simulink model "rlc_diode_sps_sl"  (R2014a)
settings: Solver=ode23tb  StartTime=0.0  StopTime=1  MaxStep=0.1  RelTol=1e-4
PreLoadFcn:
  | Vs = 30;
  | L = 1e-3;
  | C = 1e-3;
  | R = 1;
  | sys=power_analyze('rlc_diode_sps','structure');
libraries: powerlib x9
settings Model: Creator=gdudgeon  LastModifiedBy=cosorio
settings DataIOCC: SignalLoggingSaveFormat=ModelDataLogs  SaveTime=off
settings OptimizationCC: ExpressionDepthLimit=2147483647
settings DebuggingCC: UnderspecifiedInitializationDetection=Classic  FcnCallInpInsideContextMsg=UseLocalSettings  StateNameClashWarn=warning
settings GRTTargetCC: CombineOutputUpdateFcns=off  GRTInterface=on

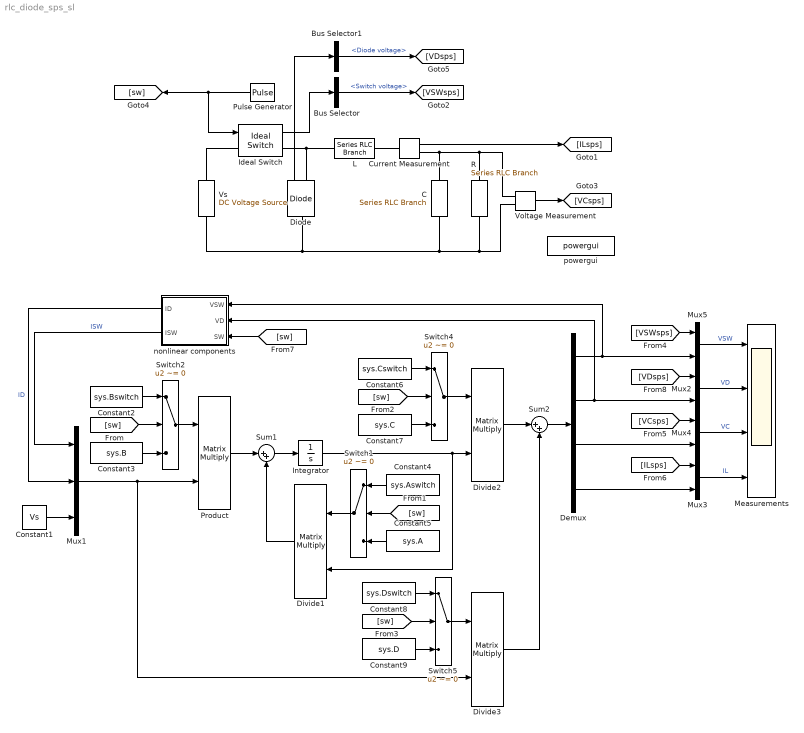
== system rlc_diode_sps_sl ==
  Bus Selector : BusSelector  OutputSignals=Switch voltage
  Bus Selector1 : BusSelector  OutputSignals=Diode voltage
  C : powerlib/Elements/Series RLC Branch  LConnTagsString=__new0  RConnTagsString=__new0  BranchType=C  Resistance=R  Inductance=1e-3  SetiL0=off  InitialCurrent=0  Capacitance=C  Setx0=off  InitialVoltage=0  Measurements=None
  Constant1 : Constant  Value=Vs
  Constant2 : Constant  Value=sys.Bswitch  VectorParams1D=off
  Constant3 : Constant  Value=sys.B  VectorParams1D=off
  Constant4 : Constant  Value=sys.Aswitch
  Constant5 : Constant  Value=sys.A
  Constant6 : Constant  Value=sys.Cswitch
  Constant7 : Constant  Value=sys.C
  Constant8 : Constant  Value=sys.Dswitch
  Constant9 : Constant  Value=sys.D
  Current Measurement : powerlib/Measurements/Current Measurement  PhasorSimulation=off  OutputType=Complex  PSBequivalent=0
  Demux : Demux
  Diode : powerlib/Power Electronics/Diode  Ron=0.001  Lon=0  Vf=0  IC=0  UseSnubber=off  Rs=1e5  Cs=Inf  Measurements=on
  Divide1 : Product  Multiplication=Matrix(*)
  Divide2 : Product  Multiplication=Matrix(*)
  Divide3 : Product  Multiplication=Matrix(*)
  Ideal Switch : powerlib/Power Electronics/Ideal Switch  Ron=0.001  Lon=0  IC=1  Rs=1e5  Cs=inf  Measurements=on
  Integrator : Integrator  InitialCondition=sys.x0
  L : powerlib/Elements/Series RLC Branch  LConnTagsString=__new0  RConnTagsString=__new0  BranchType=L  Resistance=1  Inductance=L  SetiL0=off  InitialCurrent=0  Capacitance=1e-6  Setx0=off  InitialVoltage=0  Measurements=None
  Measurements : Scope  NumInputPorts=4
      settings: YMin=0~-40~0~0  YMax=40~0~20~20
  Mux1 : Mux  Inputs=3
  Mux{2..5} (4 alike) : Mux  Inputs=2
  Product : Product  Multiplication=Matrix(*)  RndMeth=Zero
  Pulse Generator : DiscretePulseGenerator  PulseType=Time based  Period=1e-3  PulseWidth=50
  R : powerlib/Elements/Series RLC Branch  LConnTagsString=__new0  RConnTagsString=__new0  BranchType=R  Resistance=R  Inductance=1e-3  SetiL0=off  InitialCurrent=0  Capacitance=1e-6  Setx0=off  InitialVoltage=0  Measurements=None
  Sum1 : Sum  Inputs=|++
  Sum2 : Sum  Inputs=|++
  Switch{1..2,4..5} (4 alike) : Switch  Criteria=u2 ~= 0  Threshold=0.5
  Voltage Measurement : powerlib/Measurements/Voltage Measurement  PhasorSimulation=off  OutputType=Complex  PSBequivalent=0
  Vs : powerlib/Electrical Sources/DC Voltage Source  Amplitude=Vs  Measurements=None
  nonlinear components : Subsystem
  powergui : powerlib/powergui  SimulationMode=Continuous  SolverType=Tustin  SampleTime=50e-6  frequency=60  SPID=off  DisableSnubberDevices=off  DisableRonSwitches=off  DisableVfSwitches=off  SwTol=0  Interpol=off  DisplayEquations=off  Ts=0  methode=off  frequencyindice=0  Pbase=100e6  ErrMax=1e-4  Iterations=50  UnitsV=kV  UnitsW=MW  FunctionMessages=off  echomessages=off  HookPort=off  EnableUseOfTLC=off  x0status=blocks  RestoreLinks=warning  ResistiveCurrentMeasurement=off  Frange=[0:2:500]  Ylog=off  Xlog=on  ShowGrid=off  save=off  variable=ZData  structure=0  ZoomFFT=on  StartTime=0.0  cycles=1  DisplayStyle=1  fundamental=60  FreqAxis=off  MaxFrequency=1000  frequencyindicesteady=1  RmsSteady=1  display=off
  wires:
  Current Measurement/1 -> [ILsps]
  Voltage Measurement/1 -> [VCsps]
  Pulse Generator/1 -> Ideal Switch/1, [sw]
  Sum2/1 -> Demux/1
  Product/1 -> Sum1/1
  Sum1/1 -> Integrator/1
  Integrator/1 -> Divide2/2, Divide1/2
  [sw] -> Switch1/2
  Constant4/1 -> Switch1/1
  Constant5/1 -> Switch1/3
  [sw] -> Switch4/2
  Constant7/1 -> Switch4/3
  Switch4/1 -> Divide2/1
  Divide2/1 -> Sum2/1
  Divide3/1 -> Sum2/2
  [sw] -> Switch5/2
  Constant8/1 -> Switch5/1
  Constant9/1 -> Switch5/3
  Switch5/1 -> Divide3/1
  nonlinear components/2(ISW) -> Mux1/1  "ISW"
  Constant6/1 -> Switch4/1
  Demux/1 -> Mux5/2, nonlinear components/1(VSW)
  [VSWsps] -> Mux5/1
  [VCsps] -> Mux4/1
  [ILsps] -> Mux3/1
  Mux1/1 -> Product/2, Divide3/2
  Constant3/1 -> Switch2/3
  Switch2/1 -> Product/1
  Constant2/1 -> Switch2/1
  [sw] -> Switch2/2
  Mux5/1 -> Measurements/1  "VSW"
  Divide1/1 -> Sum1/2
  Switch1/1 -> Divide1/1
  Ideal Switch/1 -> Bus Selector/1
  Bus Selector/1 -> [VSWsps]  "<Switch voltage>"
  Constant1/1 -> Mux1/3
  nonlinear components/1(ID) -> Mux1/2  "ID"
  Demux/4 -> Mux3/2
  Demux/3 -> Mux4/2
  Mux3/1 -> Measurements/4  "IL"
  Mux4/1 -> Measurements/3  "VC"
  Mux2/1 -> Measurements/2  "VD"
  [VDsps] -> Mux2/1
  Demux/2 -> nonlinear components/2(VD), Mux2/2
  Diode/1 -> Bus Selector1/1
  Bus Selector1/1 -> [VDsps]  "<Diode voltage>"
  [sw] -> nonlinear components/3(SW)
  connections:
  L/RConn1 -- Current Measurement/LConn1
  Current Measurement/RConn1 -- C/LConn1 -- R/LConn1 -- Voltage Measurement/LConn1
  R/RConn1 -- Voltage Measurement/LConn2 -- C/RConn1 -- Vs/LConn1 -- Diode/LConn1
  Ideal Switch/RConn1 -- L/LConn1 -- Diode/RConn1
  Ideal Switch/LConn1 -- Vs/RConn1

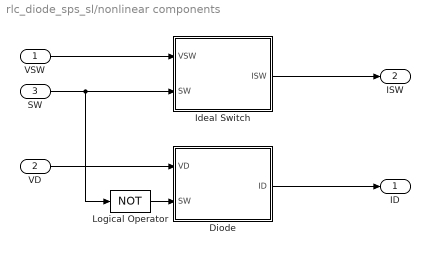
== system rlc_diode_sps_sl/nonlinear components ==
  VSW : Inport
  VD : Inport  Port=2
  SW : Inport  Port=3
  Diode : Subsystem
  Ideal Switch : Subsystem
  Logical Operator : Logic  Operator=NOT  AllPortsSameDT=off  OutDataTypeStr=boolean
  ID : Outport
  ISW : Outport  Port=2
  wires:
  VSW/1 -> Ideal Switch/1(VSW)
  SW/1 -> Logical Operator/1, Ideal Switch/2(SW)
  Ideal Switch/1(ISW) -> ISW/1
  VD/1 -> Diode/1(VD)
  Diode/1(ID) -> ID/1
  Logical Operator/1 -> Diode/2(SW)

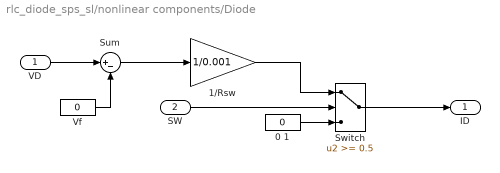
== system rlc_diode_sps_sl/nonlinear components/Diode ==
  VD : Inport
  SW : Inport  Port=2
  0 1 : Constant  Value=0
  1/Rsw : Gain  Gain=1/0.001  SaturateOnIntegerOverflow=on  OutDataTypeStr=Inherit: Same as input  ParamDataTypeStr=Inherit: Same as input
  Sum : Sum  Inputs=|+-
  Switch : Switch  Threshold=0.5  InputSameDT=on
  Vf : Constant  Value=0
  ID : Outport
  wires:
  Switch/1 -> ID/1
  1/Rsw/1 -> Switch/1
  0 1/1 -> Switch/3
  SW/1 -> Switch/2
  Sum/1 -> 1/Rsw/1
  VD/1 -> Sum/1
  Vf/1 -> Sum/2

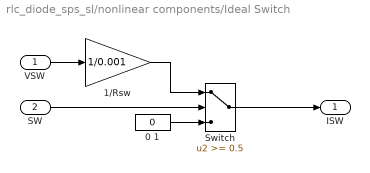
== system rlc_diode_sps_sl/nonlinear components/Ideal Switch ==
  VSW : Inport
  SW : Inport  Port=2
  0 1 : Constant  Value=0
  1/Rsw : Gain  Gain=1/0.001  SaturateOnIntegerOverflow=on  OutDataTypeStr=Inherit: Same as input  ParamDataTypeStr=Inherit: Same as input
  Switch : Switch  Threshold=0.5  InputSameDT=on
  ISW : Outport
  wires:
  SW/1 -> Switch/2
  0 1/1 -> Switch/3
  1/Rsw/1 -> Switch/1
  VSW/1 -> 1/Rsw/1
  Switch/1 -> ISW/1
